simulink model "plain_FES"  (R2021a)
settings: Solver=VariableStepAuto  StartTime=0.0  StopTime=60.0  RelTol=1e-3
values from neighbouring files (symbols this model uses):
  beta = 0.6    [FES_setup.m]
  C = [0.165, 0.05, 0.09, 0.18, 0.11, 0.04, 0.06, 0.028, 0.09]    [FES_setup.m]
  f = [30,30,30,30,30,30,30,30,30]    [FES_setup.m]
  fit_min = [0, 0, 0.2, 0.2, 0, 0, 0, 0.5, 0.3]    [FES_setup.m]
  Fmax = 0.45*[1850, 2370, 2190, 400, 1000, 5200, 1600, 3600, 1100]    [FES_setup.m]
  lopt = [0.146, 0.11, 0.121, 0.173, 0.086, 0.086, 0.054, 0.033, 0.099]    [FES_setup.m]
  Mvis = [ 2.0 1.0 0.6]    [FES_setup.m]
  Tca = [0.04, 0.04, 0.05, 0.05, 0.03, 0.04, 0.05, 0.07, 0.06]    [FES_setup.m]
  Tdel = 0.025    [FES_setup.m]
  Tfat = [18, 18, 25, 25, 18, 18, 18, 40, 33]    [FES_setup.m]
  Trec = 30    [FES_setup.m]
  vm = [0.73, 0.54, 0.48, 0.69, 0.51, 0.48, 0.32, 0.1, 0.36]    [FES_setup.m]
settings Model: Creator=nathanielgoldfarb  LastModifiedBy=nathanielgoldfarb

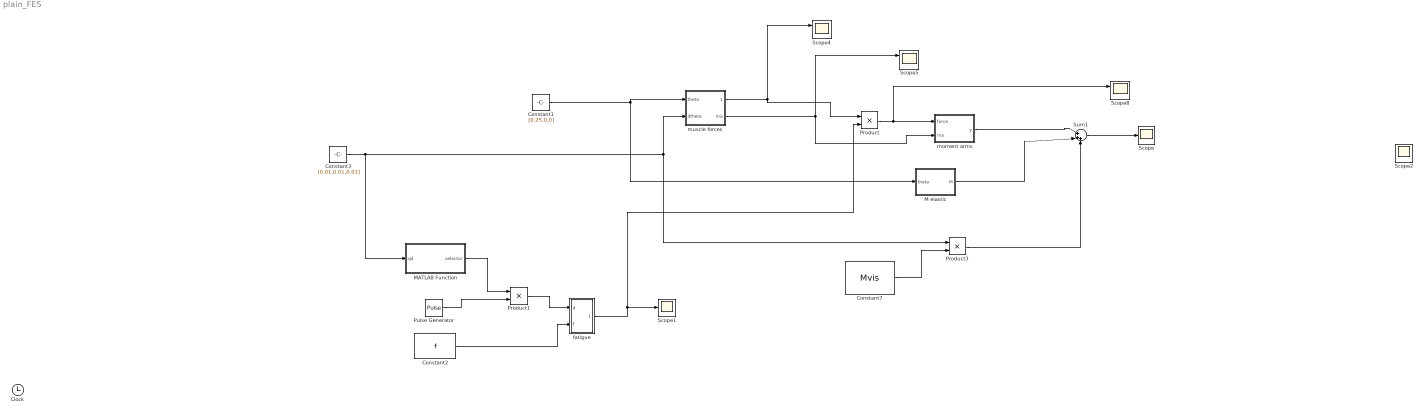
== system plain_FES ==
  Clock : Clock
  Constant1 : Constant  Value=[0.25,0,0]
  Constant2 : Constant  Value=f
  Constant3 : Constant  Value=[0.01,0.01,0.01]
  Constant7 : Constant  Value=Mvis
  M elastic : MATLAB Function  TreatAsAtomicUnit=on
  MATLAB Function : MATLAB Function  TreatAsAtomicUnit=on
  Product : Product
  Product1 : Product
  Product3 : Product
  Pulse Generator : DiscretePulseGenerator  PulseType=Time based  Amplitude=500  Period=0.5  PulseWidth=50
  Scope : Scope
  Scope1 : Scope
  Scope{2,4..5,8} (4 alike) : Scope  NumInputPorts=2
  Sum1 : Sum  Inputs=|+++
  fatigue : Subsystem
  moment arms : MATLAB Function  TreatAsAtomicUnit=on
  muscle forces : Subsystem
  wires:
  moment arms/1(y) -> Sum1/1
  Sum1/1 -> Scope/1
  Product3/1 -> Sum1/3
  M elastic/1(M) -> Sum1/2
  Product/1 -> Scope8/1, moment arms/1(force)
  Constant2/1 -> fatigue/2(f)
  Constant7/1 -> Product3/2
  fatigue/1(pulse) -> Product/2, Scope1/1
  Constant1/1 -> M elastic/1(theta), muscle forces/1(theta)
  Constant3/1 -> MATLAB Function/1(qd), Product3/1, muscle forces/2(dtheta)
  muscle forces/1(muscle) -> Product/1, Scope4/1
  muscle forces/2(ma) -> moment arms/2(ma), Scope5/1
  Pulse Generator/1 -> Product1/2
  Product1/1 -> fatigue/1(d)
  MATLAB Function/1(selector) -> Product1/1

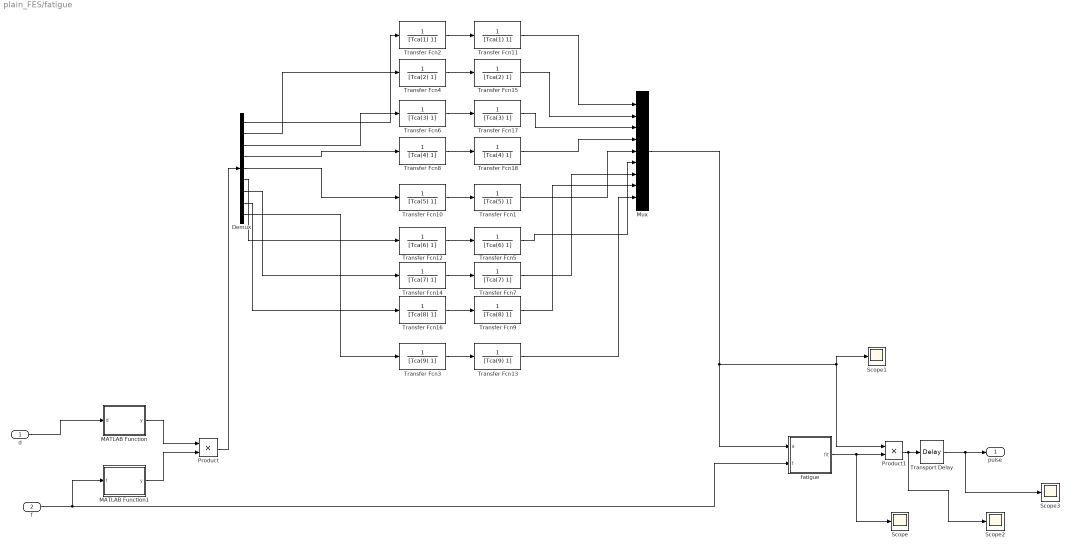
== system plain_FES/fatigue ==
  d : Inport
  f : Inport  Port=2
  Demux : Demux  Outputs=9
  MATLAB Function : MATLAB Function  TreatAsAtomicUnit=on
  MATLAB Function1 : MATLAB Function  TreatAsAtomicUnit=on
  Mux : Mux  Inputs=9
  Product : Product
  Product1 : Product
  Scope{,1..3} (4 alike) : Scope
  Transfer Fcn1 : TransferFcn  Denominator=[Tca(5) 1]
  Transfer Fcn10 : TransferFcn  Denominator=[Tca(5) 1]
  Transfer Fcn11 : TransferFcn  Denominator=[Tca(1) 1]
  Transfer Fcn12 : TransferFcn  Denominator=[Tca(6) 1]
  Transfer Fcn13 : TransferFcn  Denominator=[Tca(9) 1]
  Transfer Fcn14 : TransferFcn  Denominator=[Tca(7) 1]
  Transfer Fcn15 : TransferFcn  Denominator=[Tca(2) 1]
  Transfer Fcn16 : TransferFcn  Denominator=[Tca(8) 1]
  Transfer Fcn17 : TransferFcn  Denominator=[Tca(3) 1]
  Transfer Fcn18 : TransferFcn  Denominator=[Tca(4) 1]
  Transfer Fcn2 : TransferFcn  Denominator=[Tca(1) 1]
  Transfer Fcn3 : TransferFcn  Denominator=[Tca(9) 1]
  Transfer Fcn4 : TransferFcn  Denominator=[Tca(2) 1]
  Transfer Fcn5 : TransferFcn  Denominator=[Tca(6) 1]
  Transfer Fcn6 : TransferFcn  Denominator=[Tca(3) 1]
  Transfer Fcn7 : TransferFcn  Denominator=[Tca(7) 1]
  Transfer Fcn8 : TransferFcn  Denominator=[Tca(4) 1]
  Transfer Fcn9 : TransferFcn  Denominator=[Tca(8) 1]
  Transport Delay : TransportDelay  DelayTime=Tdel
  fatigue : Subsystem
  pulse : Outport
  wires:
  fatigue/1(fit) -> Scope/1, Product1/2
  f/1 -> MATLAB Function1/1(f), fatigue/2(f)
  Transport Delay/1 -> Scope3/1, pulse/1
  d/1 -> MATLAB Function/1(d)
  Product1/1 -> Transport Delay/1, Scope2/1
  MATLAB Function/1(y) -> Product/1
  MATLAB Function1/1(y) -> Product/2
  Demux/2 -> Transfer Fcn4/1
  Transfer Fcn8/1 -> Transfer Fcn18/1
  Demux/7 -> Transfer Fcn14/1
  Demux/6 -> Transfer Fcn12/1
  Demux/9 -> Transfer Fcn3/1
  Demux/3 -> Transfer Fcn6/1
  Transfer Fcn6/1 -> Transfer Fcn17/1
  Demux/8 -> Transfer Fcn16/1
  Demux/1 -> Transfer Fcn2/1
  Demux/5 -> Transfer Fcn10/1
  Transfer Fcn4/1 -> Transfer Fcn15/1
  Transfer Fcn10/1 -> Transfer Fcn1/1
  Transfer Fcn16/1 -> Transfer Fcn9/1
  Transfer Fcn3/1 -> Transfer Fcn13/1
  Transfer Fcn14/1 -> Transfer Fcn7/1
  Demux/4 -> Transfer Fcn8/1
  Transfer Fcn2/1 -> Transfer Fcn11/1
  Transfer Fcn12/1 -> Transfer Fcn5/1
  Transfer Fcn18/1 -> Mux/4
  Transfer Fcn7/1 -> Mux/7
  Transfer Fcn17/1 -> Mux/3
  Transfer Fcn5/1 -> Mux/6
  Transfer Fcn11/1 -> Mux/1
  Transfer Fcn13/1 -> Mux/9
  Transfer Fcn15/1 -> Mux/2
  Transfer Fcn9/1 -> Mux/8
  Transfer Fcn1/1 -> Mux/5
  Product/1 -> Demux/1
  Mux/1 -> Product1/1, Scope1/1, fatigue/1(a)

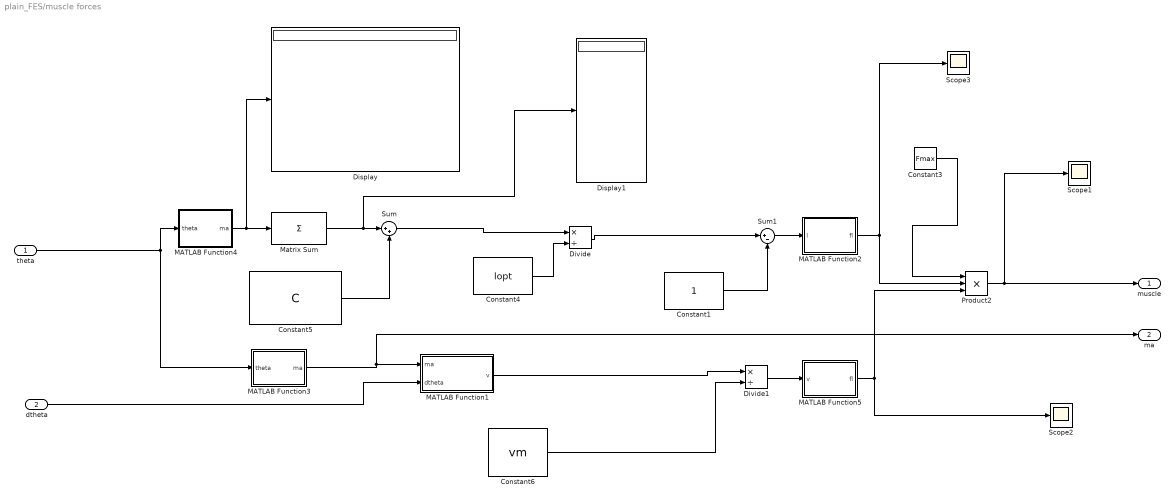
== system plain_FES/muscle forces ==
  theta : Inport
  dtheta : Inport  Port=2
  Constant1 : Constant
  Constant3 : Constant  Value=Fmax
  Constant4 : Constant  Value=lopt
  Constant5 : Constant  Value=C
  Constant6 : Constant  Value=vm
  Display : Display
  Display1 : Display
  Divide : Product  Inputs=*/
  Divide1 : Product  Inputs=*/
  MATLAB Function1 : MATLAB Function  TreatAsAtomicUnit=on
  MATLAB Function2 : MATLAB Function  TreatAsAtomicUnit=on
  MATLAB Function3 : MATLAB Function  TreatAsAtomicUnit=on
  MATLAB Function4 : MATLAB Function  TreatAsAtomicUnit=on
  MATLAB Function5 : MATLAB Function  TreatAsAtomicUnit=on
  Matrix Sum : Sum  Inputs=+  CollapseMode=Specified dimension  CollapseDim=2
  Product2 : Product  Inputs=3
  Scope1 : Scope
  Scope2 : Scope
  Scope3 : Scope
  Sum : Sum  Inputs=|++
  Sum1 : Sum  Inputs=|+-
  muscle : Outport
  ma : Outport  Port=2
  wires:
  Constant3/1 -> Product2/1
  Constant4/1 -> Divide/2
  theta/1 -> MATLAB Function4/1(theta), MATLAB Function3/1(theta)
  Constant6/1 -> Divide1/2
  MATLAB Function3/1(ma) -> MATLAB Function1/1(ma), ma/1
  dtheta/1 -> MATLAB Function1/2(dtheta)
  Constant5/1 -> Sum/2
  Product2/1 -> Scope1/1, muscle/1
  Divide1/1 -> MATLAB Function5/1(v)
  MATLAB Function1/1(v) -> Divide1/1
  Sum/1 -> Divide/1
  Divide/1 -> Sum1/1
  Sum1/1 -> MATLAB Function2/1(l)
  Constant1/1 -> Sum1/2
  MATLAB Function4/1(ma) -> Display/1, Matrix Sum/1
  MATLAB Function5/1(fl) -> Product2/3, Scope2/1
  MATLAB Function2/1(fl) -> Scope3/1, Product2/2
  Matrix Sum/1 -> Display1/1, Sum/1

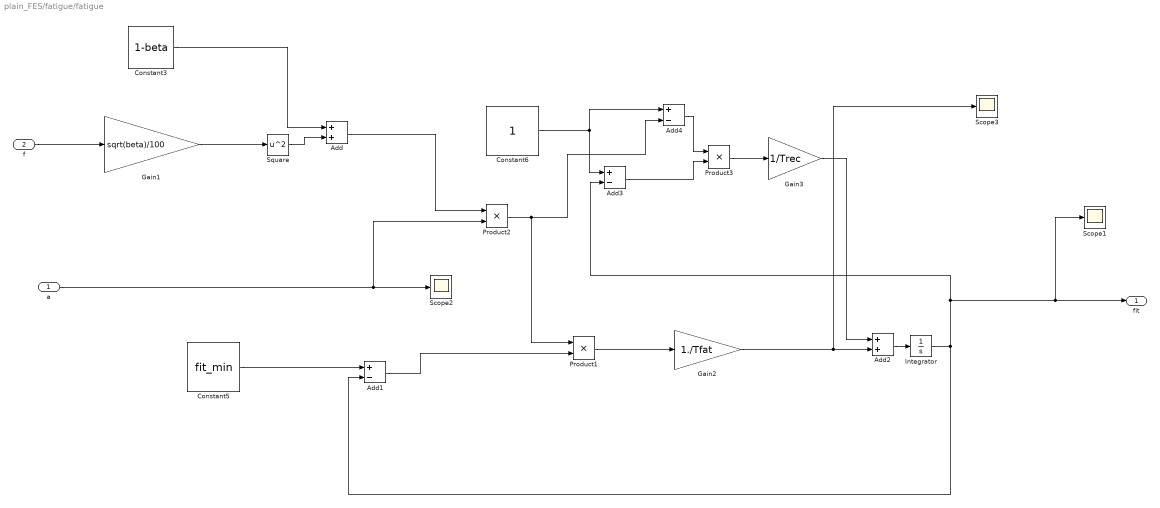
== system plain_FES/fatigue/fatigue ==
  a : Inport
  f : Inport  Port=2
  Add : Sum
  Add1 : Sum  Inputs=+-
  Add2 : Sum
  Add3 : Sum  Inputs=+-
  Add4 : Sum  Inputs=+-
  Constant3 : Constant  Value=1-beta
  Constant5 : Constant  Value=fit_min
  Constant6 : Constant
  Gain1 : Gain  Gain=sqrt(beta)/100
  Gain2 : Gain  Gain=1./Tfat
  Gain3 : Gain  Gain=1/Trec
  Integrator : Integrator  InitialCondition=1
  Product1 : Product
  Product2 : Product
  Product3 : Product
  Scope1 : Scope
  Scope2 : Scope
  Scope3 : Scope
  Square : Math  Operator=square  SaturateOnIntegerOverflow=on
  fit : Outport
  wires:
  Add4/1 -> Product3/1
  f/1 -> Gain1/1
  Product2/1 -> Product1/1, Add4/2
  Constant5/1 -> Add1/1
  Constant6/1 -> Add3/1, Add4/1
  Add3/1 -> Product3/2
  Gain1/1 -> Square/1
  Product1/1 -> Gain2/1
  Gain3/1 -> Add2/1
  Square/1 -> Add/2
  Add2/1 -> Integrator/1
  Add/1 -> Product2/1
  Constant3/1 -> Add/1
  Add1/1 -> Product1/2
  Product3/1 -> Gain3/1
  Integrator/1 -> Add1/2, Scope1/1, fit/1, Add3/2
  a/1 -> Product2/2, Scope2/1
  Gain2/1 -> Scope3/1, Add2/2

== matlab function plain_FES/fatigue/MATLAB Function ==
  data: y output; d input
function y = fcn( d )
    
  y = recruitment( d);



end

== matlab function plain_FES/muscle forces/MATLAB Function2 ==
  data: l input; fl output
function fl = fcn(l)

    fl = force_length(l);

end

== matlab function plain_FES/muscle forces/MATLAB Function3 ==
  data: theta input; ma output
function ma = fcn(theta)

    ma = calc_ma(theta);
end

== matlab function plain_FES/muscle forces/MATLAB Function4 ==
  data: theta input; ma output
function ma  = fcn(theta)

    ma = dma(theta);
end

== matlab function plain_FES/muscle forces/MATLAB Function5 ==
  data: v input; fl output
function fl = fcn(v)

    fl = force_velocity(v);

end

== matlab function plain_FES/moment arms ==
  data: force input; y output; ma input
function y = fcn(force, ma)

y = moment_calc(force, ma);

== matlab function plain_FES/M elastic ==
  data: theta input; M output
function M = fcn(theta)

    hip = theta(1);
    knee = theta(2);
    ankle = theta(3);
    
    M_H = exp(2.1080 - 0.0160*knee - 0.0195*hip) - exp(-2.1784 + 0.070*knee + 0.1349*hip) - 15.24;
    
    M_K = exp(1.0372 + 0.0040*ankle - 0.0494*knee - 0.0250*hip)-...
          exp(-1.1561 - 0.0020*ankle + 0.0254*knee + 0.0030*hip)+...
          exp(2.5-0.25*knee) + 1.0;
    
      M_A = exp(2.0111 - 0.0833*ankle - 0.0090)-...
          exp(-9.9250 + 0.2132*ankle) - 2.970;
    
      
    M = [ M_H, M_K, M_A];

end

== matlab function plain_FES/muscle forces/MATLAB Function1 ==
  data: ma input; v output; dtheta input
function v = fcn(ma, dtheta)

  v = zeros(9,1);
    for ii = 1:3
      for jj = 1:9
          v(jj) = v(jj) + dtheta(ii) * ma(jj,ii);
      end
    end

end

== matlab function plain_FES/MATLAB Function ==
  data: qd input; selector output
function selector = fcn(qd)


    selector = zeros(9,1);

    hip_sign = sign(qd(1));
    knee_sign = sign(qd(2));
    ankle_sign = sign(qd(3));
    
    
    if hip == 1
        selector(1) = 1;
    elseif hip == -1
        selector(2) = 1;
        selector(3) = 1;
    end
    
    if knee == 1
        selector(6) = 1;
    elseif knee == -1
        selector(4) = 1;
    end
    
    if ankle == 1
        selector(9) = 1;
    elseif hip == -1
        selector(8) = 1;
    end
    

    if hip && knee == 1
        selector(5) = 1;
    end
    
    
    if hip && knee == -1
        selector(7) = 1;
    end
    
end

== matlab function plain_FES/fatigue/MATLAB Function1 ==
  data: f input; y output
function y = fcn(f )

  y = frequencyChar(f);



end
